simulink subsystem "AeroPropRefFranc"  (R2024b)
settings: Solver=VariableStepAuto  StartTime=0.0  StopTime=10.0  RelTol=1e-3
undefined symbols (not defined in the file or in its folder): ess, Force_b, Fprop_r, geom, H_b, Hdot_b, Moment_b, mot, mot2, mot3, mot4, Mprop_r, propel, propel2, propel3, propel4, pxf_diagram_options, SimIn, SimPar, tc, tc2, tc3, tc4
libraries: simulink x8, slpidlib x4, starslibAxisTransformations x2, libAxisTransformations x2
(part 3 of 10)

== system AeroPropRefFranc/Propulsion and Aerodynamic Forces and Moments/S-Function/Battery Model/powerplant/mot4/plant ==
  aInport--1 : Inport
  inport-ctrl_bus-2 : Inport  Port=2
  in-effort-2 : Inport  Port=3
  in-flow-3 : Inport  Port=4
  Ground_1 : Ground
  Terminator_1 : Terminator
  mot4_plant_map_Pelec_funTW_volt_in : Subsystem
  parameter_out : Subsystem
  parameter_selection : Subsystem
  outport-system_info_bus : Outport
  outport-plant_bus : Outport  Port=2
  out-effort-7 : Outport  Port=3
  out-flow-8 : Outport  Port=4
  wires:
  Ground_1/1 -> parameter_selection/1(Inport_1)
  aInport--1/1 -> Terminator_1/1
  mot4_plant_map_Pelec_funTW_volt_in/8(mot_current_out) -> out-flow-8/1
  mot4_plant_map_Pelec_funTW_volt_in/7(mot_trq_out mot_inertia_out) -> out-effort-7/1
  in-flow-3/1 -> mot4_plant_map_Pelec_funTW_volt_in/3(spd)
  in-effort-2/1 -> mot4_plant_map_Pelec_funTW_volt_in/2(voltage)
  parameter_selection/1(outport-mot4_ctrl_cmd_simu-1) -> mot4_plant_map_Pelec_funTW_volt_in/1(mot_ctrl_cmd_simu)
  mot4_plant_map_Pelec_funTW_volt_in/6(mot_plant_temp_coeff_simu) -> parameter_out/6(inport-mot4_plant_temp_coeff_simu)
  mot4_plant_map_Pelec_funTW_volt_in/5(mot_plant_trq_out_simu) -> parameter_out/5(inport-mot4_plant_trq_out_simu)
  mot4_plant_map_Pelec_funTW_volt_in/4(mot_plant_cmd_simu) -> parameter_out/4(inport-mot4_plant_cmd_simu)
  mot4_plant_map_Pelec_funTW_volt_in/3(mot_plant_volt_in_simu) -> parameter_out/3(inport-mot4_plant_volt_in_simu)
  mot4_plant_map_Pelec_funTW_volt_in/2(mot_plant_curr_in_simu) -> parameter_out/2(inport-mot4_plant_curr_in_simu)
  mot4_plant_map_Pelec_funTW_volt_in/1(mot_plant_spd_out_simu) -> parameter_out/1(inport-mot4_plant_spd_out_simu)
  parameter_out/2(outport-plant_bus) -> outport-plant_bus/1
  parameter_out/1(outport-system_info_bus) -> outport-system_info_bus/1
  inport-ctrl_bus-2/1 -> parameter_selection/2(inport-ctrl_bus-2)

== system AeroPropRefFranc/Propulsion and Aerodynamic Forces and Moments/S-Function/Battery Model/powerplant/propel/plant ==
  inport-main_info_bus-1 : Inport
  aInport--2 : Inport  Port=2
  in-effort-4 : Inport  Port=3
  in-flow-5 : Inport  Port=4
  Ground_1 : Ground
  Terminator_1 : Terminator
  parameter_out : Subsystem
  parameter_selection : Subsystem
  propel_plant_uas : Subsystem
  outport-system_info_bus : Outport
  aOutport--2 : Outport  Port=2
  out-effort-5 : Outport  Port=3
  out-flow-6 : Outport  Port=4
  wires:
  Ground_1/1 -> aOutport--2/1
  aInport--2/1 -> Terminator_1/1
  propel_plant_uas/6(propel_plant_speed_out_simu) -> out-flow-6/1
  propel_plant_uas/5(propel_plant_effort) -> out-effort-5/1
  in-flow-5/1 -> propel_plant_uas/5(flow-in)
  in-effort-4/1 -> propel_plant_uas/4(tc_plant_trq_out_simu)
  parameter_selection/3(outport-eqnmotion_plant_linvel_simu-3) -> propel_plant_uas/3(eqnmotion_plant_linvel_simu)
  parameter_selection/2(outport-tc_plant_inertia_out_simu-2) -> propel_plant_uas/2(tc_plant_inertia_out_simu)
  parameter_selection/1(outport-env_plant_density_simu-1) -> propel_plant_uas/1(env_plant_density_simu)
  propel_plant_uas/4(propel_plant_thrust_simu) -> parameter_out/4(inport-propel_plant_thrust_simu)
  propel_plant_uas/3(propel_plant_pwr_out_simu) -> parameter_out/3(inport-propel_plant_pwr_out_simu)
  propel_plant_uas/2(propel_plant_pwr_in_simu) -> parameter_out/2(inport-propel_plant_pwr_in_simu)
  propel_plant_uas/1(propel_plant_speed_simu) -> parameter_out/1(inport-propel_plant_speed_simu)
  parameter_out/1(outport-system_info_bus) -> outport-system_info_bus/1
  inport-main_info_bus-1/1 -> parameter_selection/1(inport-main_info_bus-1)

== system AeroPropRefFranc/Propulsion and Aerodynamic Forces and Moments/S-Function/Battery Model/powerplant/propel2/plant ==
  inport-main_info_bus-1 : Inport
  aInport--2 : Inport  Port=2
  in-effort-4 : Inport  Port=3
  in-flow-5 : Inport  Port=4
  Ground_1 : Ground
  Terminator_1 : Terminator
  parameter_out : Subsystem
  parameter_selection : Subsystem
  propel2_plant_uas : Subsystem
  outport-system_info_bus : Outport
  aOutport--2 : Outport  Port=2
  out-effort-5 : Outport  Port=3
  out-flow-6 : Outport  Port=4
  wires:
  Ground_1/1 -> aOutport--2/1
  aInport--2/1 -> Terminator_1/1
  propel2_plant_uas/6(propel_plant_speed_out_simu) -> out-flow-6/1
  propel2_plant_uas/5(propel_plant_effort) -> out-effort-5/1
  in-flow-5/1 -> propel2_plant_uas/5(flow-in)
  in-effort-4/1 -> propel2_plant_uas/4(tc_plant_trq_out_simu)
  parameter_selection/3(outport-eqnmotion_plant_linvel_simu-3) -> propel2_plant_uas/3(eqnmotion_plant_linvel_simu)
  parameter_selection/2(outport-tc_plant_inertia_out_simu-2) -> propel2_plant_uas/2(tc_plant_inertia_out_simu)
  parameter_selection/1(outport-env_plant_density_simu-1) -> propel2_plant_uas/1(env_plant_density_simu)
  propel2_plant_uas/4(propel_plant_thrust_simu) -> parameter_out/4(inport-propel2_plant_thrust_simu)
  propel2_plant_uas/3(propel_plant_pwr_out_simu) -> parameter_out/3(inport-propel2_plant_pwr_out_simu)
  propel2_plant_uas/2(propel_plant_pwr_in_simu) -> parameter_out/2(inport-propel2_plant_pwr_in_simu)
  propel2_plant_uas/1(propel_plant_speed_simu) -> parameter_out/1(inport-propel2_plant_speed_simu)
  parameter_out/1(outport-system_info_bus) -> outport-system_info_bus/1
  inport-main_info_bus-1/1 -> parameter_selection/1(inport-main_info_bus-1)

== system AeroPropRefFranc/Propulsion and Aerodynamic Forces and Moments/S-Function/Battery Model/powerplant/propel3/plant ==
  inport-main_info_bus-1 : Inport
  aInport--2 : Inport  Port=2
  in-effort-4 : Inport  Port=3
  in-flow-5 : Inport  Port=4
  Ground_1 : Ground
  Terminator_1 : Terminator
  parameter_out : Subsystem
  parameter_selection : Subsystem
  propel3_plant_uas : Subsystem
  outport-system_info_bus : Outport
  aOutport--2 : Outport  Port=2
  out-effort-5 : Outport  Port=3
  out-flow-6 : Outport  Port=4
  wires:
  Ground_1/1 -> aOutport--2/1
  aInport--2/1 -> Terminator_1/1
  propel3_plant_uas/6(propel_plant_speed_out_simu) -> out-flow-6/1
  propel3_plant_uas/5(propel_plant_effort) -> out-effort-5/1
  in-flow-5/1 -> propel3_plant_uas/5(flow-in)
  in-effort-4/1 -> propel3_plant_uas/4(tc_plant_trq_out_simu)
  parameter_selection/3(outport-eqnmotion_plant_linvel_simu-3) -> propel3_plant_uas/3(eqnmotion_plant_linvel_simu)
  parameter_selection/2(outport-tc_plant_inertia_out_simu-2) -> propel3_plant_uas/2(tc_plant_inertia_out_simu)
  parameter_selection/1(outport-env_plant_density_simu-1) -> propel3_plant_uas/1(env_plant_density_simu)
  propel3_plant_uas/4(propel_plant_thrust_simu) -> parameter_out/4(inport-propel3_plant_thrust_simu)
  propel3_plant_uas/3(propel_plant_pwr_out_simu) -> parameter_out/3(inport-propel3_plant_pwr_out_simu)
  propel3_plant_uas/2(propel_plant_pwr_in_simu) -> parameter_out/2(inport-propel3_plant_pwr_in_simu)
  propel3_plant_uas/1(propel_plant_speed_simu) -> parameter_out/1(inport-propel3_plant_speed_simu)
  parameter_out/1(outport-system_info_bus) -> outport-system_info_bus/1
  inport-main_info_bus-1/1 -> parameter_selection/1(inport-main_info_bus-1)

== system AeroPropRefFranc/Propulsion and Aerodynamic Forces and Moments/S-Function/Battery Model/powerplant/propel4/plant ==
  inport-main_info_bus-1 : Inport
  aInport--2 : Inport  Port=2
  in-effort-4 : Inport  Port=3
  in-flow-5 : Inport  Port=4
  Ground_1 : Ground
  Terminator_1 : Terminator
  parameter_out : Subsystem
  parameter_selection : Subsystem
  propel4_plant_uas : Subsystem
  outport-system_info_bus : Outport
  aOutport--2 : Outport  Port=2
  out-effort-5 : Outport  Port=3
  out-flow-6 : Outport  Port=4
  wires:
  Ground_1/1 -> aOutport--2/1
  aInport--2/1 -> Terminator_1/1
  propel4_plant_uas/6(propel_plant_speed_out_simu) -> out-flow-6/1
  propel4_plant_uas/5(propel_plant_effort) -> out-effort-5/1
  in-flow-5/1 -> propel4_plant_uas/5(flow-in)
  in-effort-4/1 -> propel4_plant_uas/4(tc_plant_trq_out_simu)
  parameter_selection/3(outport-eqnmotion_plant_linvel_simu-3) -> propel4_plant_uas/3(eqnmotion_plant_linvel_simu)
  parameter_selection/2(outport-tc_plant_inertia_out_simu-2) -> propel4_plant_uas/2(tc_plant_inertia_out_simu)
  parameter_selection/1(outport-env_plant_density_simu-1) -> propel4_plant_uas/1(env_plant_density_simu)
  propel4_plant_uas/4(propel_plant_thrust_simu) -> parameter_out/4(inport-propel4_plant_thrust_simu)
  propel4_plant_uas/3(propel_plant_pwr_out_simu) -> parameter_out/3(inport-propel4_plant_pwr_out_simu)
  propel4_plant_uas/2(propel_plant_pwr_in_simu) -> parameter_out/2(inport-propel4_plant_pwr_in_simu)
  propel4_plant_uas/1(propel_plant_speed_simu) -> parameter_out/1(inport-propel4_plant_speed_simu)
  parameter_out/1(outport-system_info_bus) -> outport-system_info_bus/1
  inport-main_info_bus-1/1 -> parameter_selection/1(inport-main_info_bus-1)

== system AeroPropRefFranc/Propulsion and Aerodynamic Forces and Moments/S-Function/Battery Model/powerplant/tc/plant ==
  aInport--1 : Inport
  aInport--2 : Inport  Port=2
  in-effort-1 : Inport  Port=3
  in-flow-2 : Inport  Port=4
  Ground_1 : Ground
  Terminator_1 : Terminator
  Terminator_2 : Terminator
  parameter_out : Subsystem
  parameter_selection : Subsystem
  tc_plant_map_trqloss_funTW : Subsystem
  outport-system_info_bus : Outport
  aOutport--2 : Outport  Port=2
  out-effort-7 : Outport  Port=3
  out-flow-8 : Outport  Port=4
  wires:
  Ground_1/1 -> aOutport--2/1
  aInport--2/1 -> Terminator_2/1
  aInport--1/1 -> Terminator_1/1
  tc_plant_map_trqloss_funTW/8(tc_spd_in) -> out-flow-8/1
  tc_plant_map_trqloss_funTW/7(tc_trq_out) -> out-effort-7/1
  in-flow-2/1 -> tc_plant_map_trqloss_funTW/2(tc_spd_out)
  in-effort-1/1 -> tc_plant_map_trqloss_funTW/1(tc_trq_in tc_inertia_in)
  tc_plant_map_trqloss_funTW/6(tc_plant_inertia_out_simu) -> parameter_out/6(inport-tc_plant_inertia_out_simu)
  tc_plant_map_trqloss_funTW/5(tc_plant_inertia_in_simu) -> parameter_out/5(inport-tc_plant_inertia_in_simu)
  tc_plant_map_trqloss_funTW/4(tc_plant_spd_out_simu) -> parameter_out/4(inport-tc_plant_spd_out_simu)
  tc_plant_map_trqloss_funTW/3(tc_plant_spd_in_simu) -> parameter_out/3(inport-tc_plant_spd_in_simu)
  tc_plant_map_trqloss_funTW/2(tc_plant_trq_out_simu) -> parameter_out/2(inport-tc_plant_trq_out_simu)
  tc_plant_map_trqloss_funTW/1(tc_plant_trq_in_simu) -> parameter_out/1(inport-tc_plant_trq_in_simu)
  parameter_out/1(outport-system_info_bus) -> outport-system_info_bus/1

== system AeroPropRefFranc/Propulsion and Aerodynamic Forces and Moments/S-Function/Battery Model/powerplant/tc2/plant ==
  aInport--1 : Inport
  aInport--2 : Inport  Port=2
  in-effort-1 : Inport  Port=3
  in-flow-2 : Inport  Port=4
  Ground_1 : Ground
  Terminator_1 : Terminator
  Terminator_2 : Terminator
  parameter_out : Subsystem
  parameter_selection : Subsystem
  tc2_plant_map_trqloss_funTW : Subsystem
  outport-system_info_bus : Outport
  aOutport--2 : Outport  Port=2
  out-effort-7 : Outport  Port=3
  out-flow-8 : Outport  Port=4
  wires:
  Ground_1/1 -> aOutport--2/1
  aInport--2/1 -> Terminator_2/1
  aInport--1/1 -> Terminator_1/1
  tc2_plant_map_trqloss_funTW/8(tc_spd_in) -> out-flow-8/1
  tc2_plant_map_trqloss_funTW/7(tc_trq_out) -> out-effort-7/1
  in-flow-2/1 -> tc2_plant_map_trqloss_funTW/2(tc_spd_out)
  in-effort-1/1 -> tc2_plant_map_trqloss_funTW/1(tc_trq_in tc_inertia_in)
  tc2_plant_map_trqloss_funTW/6(tc_plant_inertia_out_simu) -> parameter_out/6(inport-tc2_plant_inertia_out_simu)
  tc2_plant_map_trqloss_funTW/5(tc_plant_inertia_in_simu) -> parameter_out/5(inport-tc2_plant_inertia_in_simu)
  tc2_plant_map_trqloss_funTW/4(tc_plant_spd_out_simu) -> parameter_out/4(inport-tc2_plant_spd_out_simu)
  tc2_plant_map_trqloss_funTW/3(tc_plant_spd_in_simu) -> parameter_out/3(inport-tc2_plant_spd_in_simu)
  tc2_plant_map_trqloss_funTW/2(tc_plant_trq_out_simu) -> parameter_out/2(inport-tc2_plant_trq_out_simu)
  tc2_plant_map_trqloss_funTW/1(tc_plant_trq_in_simu) -> parameter_out/1(inport-tc2_plant_trq_in_simu)
  parameter_out/1(outport-system_info_bus) -> outport-system_info_bus/1

== system AeroPropRefFranc/Propulsion and Aerodynamic Forces and Moments/S-Function/Battery Model/powerplant/tc3/plant ==
  aInport--1 : Inport
  aInport--2 : Inport  Port=2
  in-effort-1 : Inport  Port=3
  in-flow-2 : Inport  Port=4
  Ground_1 : Ground
  Terminator_1 : Terminator
  Terminator_2 : Terminator
  parameter_out : Subsystem
  parameter_selection : Subsystem
  tc3_plant_map_trqloss_funTW : Subsystem
  outport-system_info_bus : Outport
  aOutport--2 : Outport  Port=2
  out-effort-7 : Outport  Port=3
  out-flow-8 : Outport  Port=4
  wires:
  Ground_1/1 -> aOutport--2/1
  aInport--2/1 -> Terminator_2/1
  aInport--1/1 -> Terminator_1/1
  tc3_plant_map_trqloss_funTW/8(tc_spd_in) -> out-flow-8/1
  tc3_plant_map_trqloss_funTW/7(tc_trq_out) -> out-effort-7/1
  in-flow-2/1 -> tc3_plant_map_trqloss_funTW/2(tc_spd_out)
  in-effort-1/1 -> tc3_plant_map_trqloss_funTW/1(tc_trq_in tc_inertia_in)
  tc3_plant_map_trqloss_funTW/6(tc_plant_inertia_out_simu) -> parameter_out/6(inport-tc3_plant_inertia_out_simu)
  tc3_plant_map_trqloss_funTW/5(tc_plant_inertia_in_simu) -> parameter_out/5(inport-tc3_plant_inertia_in_simu)
  tc3_plant_map_trqloss_funTW/4(tc_plant_spd_out_simu) -> parameter_out/4(inport-tc3_plant_spd_out_simu)
  tc3_plant_map_trqloss_funTW/3(tc_plant_spd_in_simu) -> parameter_out/3(inport-tc3_plant_spd_in_simu)
  tc3_plant_map_trqloss_funTW/2(tc_plant_trq_out_simu) -> parameter_out/2(inport-tc3_plant_trq_out_simu)
  tc3_plant_map_trqloss_funTW/1(tc_plant_trq_in_simu) -> parameter_out/1(inport-tc3_plant_trq_in_simu)
  parameter_out/1(outport-system_info_bus) -> outport-system_info_bus/1

== system AeroPropRefFranc/Propulsion and Aerodynamic Forces and Moments/S-Function/Battery Model/powerplant/tc4/plant ==
  aInport--1 : Inport
  aInport--2 : Inport  Port=2
  in-effort-1 : Inport  Port=3
  in-flow-2 : Inport  Port=4
  Ground_1 : Ground
  Terminator_1 : Terminator
  Terminator_2 : Terminator
  parameter_out : Subsystem
  parameter_selection : Subsystem
  tc4_plant_map_trqloss_funTW : Subsystem
  outport-system_info_bus : Outport
  aOutport--2 : Outport  Port=2
  out-effort-7 : Outport  Port=3
  out-flow-8 : Outport  Port=4
  wires:
  Ground_1/1 -> aOutport--2/1
  aInport--2/1 -> Terminator_2/1
  aInport--1/1 -> Terminator_1/1
  tc4_plant_map_trqloss_funTW/8(tc_spd_in) -> out-flow-8/1
  tc4_plant_map_trqloss_funTW/7(tc_trq_out) -> out-effort-7/1
  in-flow-2/1 -> tc4_plant_map_trqloss_funTW/2(tc_spd_out)
  in-effort-1/1 -> tc4_plant_map_trqloss_funTW/1(tc_trq_in tc_inertia_in)
  tc4_plant_map_trqloss_funTW/6(tc_plant_inertia_out_simu) -> parameter_out/6(inport-tc4_plant_inertia_out_simu)
  tc4_plant_map_trqloss_funTW/5(tc_plant_inertia_in_simu) -> parameter_out/5(inport-tc4_plant_inertia_in_simu)
  tc4_plant_map_trqloss_funTW/4(tc_plant_spd_out_simu) -> parameter_out/4(inport-tc4_plant_spd_out_simu)
  tc4_plant_map_trqloss_funTW/3(tc_plant_spd_in_simu) -> parameter_out/3(inport-tc4_plant_spd_in_simu)
  tc4_plant_map_trqloss_funTW/2(tc_plant_trq_out_simu) -> parameter_out/2(inport-tc4_plant_trq_out_simu)
  tc4_plant_map_trqloss_funTW/1(tc_plant_trq_in_simu) -> parameter_out/1(inport-tc4_plant_trq_in_simu)
  parameter_out/1(outport-system_info_bus) -> outport-system_info_bus/1

== system AeroPropRefFranc/Propulsion and Aerodynamic Forces and Moments/S-Function/Battery Model/ess (battery)/ctrl/ess_ctrl_pngv_map_anl_PI_cstr/PI controller for maximal charge power and current1 ==
  ess voltage : Inport
  ess curr : Inport  Port=2
  SOC : Inport  Port=3
  Burst maximal power : Lookup  InputValues=ess.plant.init.pwr_chg_10sec.idx1_soc  Table=ess.plant.init.pwr_chg_10sec.map  SaturateOnIntegerOverflow=off
  Continuous maximal power : Lookup  InputValues=ess.plant.init.pwr_chg.idx1_soc  Table=ess.plant.init.pwr_chg.map  SaturateOnIntegerOverflow=off
  Interpolation (curr) : Fcn  Expr=u(3)*u(1) + u(2)*(1-u(1))
  Interpolation (curr)1 : Fcn  Expr=u(3)*u(1) + u(2)*(1-u(1))
  Mux1 : Mux  Inputs=3
  Mux2 : Mux  Inputs=3
  "PI Ratio Calculator (curr) " : Subsystem
  PI Ratio Calculator (curr) 1 : Subsystem
  Product : Product  RndMeth=Zero
  Saturation : Saturate  UpperLimit=0  LowerLimit=-inf
  Saturation1 : Saturate  UpperLimit=0  LowerLimit=-inf
  "ess curr " : InportShadow  Port=2
  ess maximum current (burst charge) : Lookup  InputValues=ess.plant.init.curr_chg_burst_max.idx1_soc  Table=ess.plant.init.curr_chg_burst_max.map  SaturateOnIntegerOverflow=off
  ess maximum current (continuous charge) : Lookup  InputValues=ess.plant.init.curr_chg_cont_max.idx1_soc  Table=ess.plant.init.curr_chg_cont_max.map  SaturateOnIntegerOverflow=off
  ess.init.num_cell1 : Gain  Gain=ess.plant.init.num_cell  SaturateOnIntegerOverflow=on  OutDataTypeStr=Inherit: Same as input  ParamDataTypeStr=Inherit: Same as input
  ess.init.num_cell2 : Gain  Gain=ess.plant.init.num_cell  SaturateOnIntegerOverflow=on  OutDataTypeStr=Inherit: Same as input  ParamDataTypeStr=Inherit: Same as input
  ess.init.num_module_parallel1 : Gain  Gain=ess.plant.init.num_module_parallel
  ess.init.num_module_parallel5 : Gain  Gain=ess.plant.init.num_module_parallel
  Pwr_max_reg : Outport
  Curr_max_reg : Outport  Port=2
  wires:
  Saturation/1 -> "PI Ratio Calculator (curr) "/1(ess curr)
  "PI Ratio Calculator (curr) "/1(Current ratio) -> Mux1/1
  ess maximum current (burst charge)/1 -> ess.init.num_module_parallel1/1
  ess maximum current (continuous charge)/1 -> ess.init.num_module_parallel5/1
  ess curr/1 -> Saturation/1
  Mux1/1 -> Interpolation (curr)/1
  Interpolation (curr)/1 -> Curr_max_reg/1
  SOC/1 -> Continuous maximal power/1, Burst maximal power/1, ess maximum current (continuous charge)/1, ess maximum current (burst charge)/1
  Saturation1/1 -> PI Ratio Calculator (curr) 1/1(ess pwr)
  Continuous maximal power/1 -> ess.init.num_cell2/1
  Interpolation (curr)1/1 -> Pwr_max_reg/1
  Mux2/1 -> Interpolation (curr)1/1
  PI Ratio Calculator (curr) 1/1(pwr ratio) -> Mux2/1
  Burst maximal power/1 -> ess.init.num_cell1/1
  "ess curr "/1 -> Product/2
  ess voltage/1 -> Product/1
  Product/1 -> Saturation1/1
  ess.init.num_cell2/1 -> Mux2/2, PI Ratio Calculator (curr) 1/2(pwr max cont)
  ess.init.num_cell1/1 -> Mux2/3
  ess.init.num_module_parallel5/1 -> Mux1/2, "PI Ratio Calculator (curr) "/2(curr max cont)
  ess.init.num_module_parallel1/1 -> Mux1/3

== system AeroPropRefFranc/Propulsion and Aerodynamic Forces and Moments/S-Function/Battery Model/ess (battery)/ctrl/ess_ctrl_pngv_map_anl_PI_cstr/PI controller for maximal discharge power and current1 ==
  ess voltage : Inport
  ess curr : Inport  Port=2
  SOC : Inport  Port=3
  Burst maximal power : Lookup  InputValues=ess.plant.init.pwr_dis_10sec.idx1_soc  Table=ess.plant.init.pwr_dis_10sec.map  SaturateOnIntegerOverflow=off
  Continuous maximal power : Lookup  InputValues=ess.plant.init.pwr_dis.idx1_soc  Table=ess.plant.init.pwr_dis.map  SaturateOnIntegerOverflow=off
  Interpolation (curr) : Fcn  Expr=u(3)*u(1) + u(2)*(1-u(1))
  Interpolation (curr)1 : Fcn  Expr=u(3)*u(1) + u(2)*(1-u(1))
  Mux1 : Mux  Inputs=3
  Mux2 : Mux  Inputs=3
  "PI Ratio Calculator (curr) " : Subsystem
  PI Ratio Calculator (curr) 1 : Subsystem
  Product : Product  RndMeth=Zero
  Saturation : Saturate  UpperLimit=inf  LowerLimit=0
  Saturation1 : Saturate  UpperLimit=inf  LowerLimit=0
  "ess curr " : InportShadow  Port=2
  ess maximum current (burst discharge)1 : Lookup  InputValues=ess.plant.init.curr_dis_burst_max.idx1_soc  Table=ess.plant.init.curr_dis_burst_max.map  SaturateOnIntegerOverflow=off
  "ess maximum current (continuous discharge) " : Lookup  InputValues=ess.plant.init.curr_dis_cont_max.idx1_soc  Table=ess.plant.init.curr_dis_cont_max.map  SaturateOnIntegerOverflow=off
  ess.init.num_cell1 : Gain  Gain=ess.plant.init.num_cell  SaturateOnIntegerOverflow=on  OutDataTypeStr=Inherit: Same as input  ParamDataTypeStr=Inherit: Same as input
  ess.init.num_cell2 : Gain  Gain=ess.plant.init.num_cell  SaturateOnIntegerOverflow=on  OutDataTypeStr=Inherit: Same as input  ParamDataTypeStr=Inherit: Same as input
  ess.init.num_module_parallel1 : Gain  Gain=ess.plant.init.num_module_parallel
  ess.init.num_module_parallel5 : Gain  Gain=ess.plant.init.num_module_parallel
  Curr_max_prop : Outport
  Pwr_max_prop : Outport  Port=2
  wires:
  Interpolation (curr)/1 -> Curr_max_prop/1
  Mux1/1 -> Interpolation (curr)/1
  ess curr/1 -> Saturation/1
  "ess maximum current (continuous discharge) "/1 -> ess.init.num_module_parallel5/1
  ess maximum current (burst discharge)1/1 -> ess.init.num_module_parallel1/1
  "PI Ratio Calculator (curr) "/1(Current ratio) -> Mux1/1
  Saturation/1 -> "PI Ratio Calculator (curr) "/1(ess curr)
  SOC/1 -> Continuous maximal power/1, Burst maximal power/1, "ess maximum current (continuous discharge) "/1, ess maximum current (burst discharge)1/1
  Saturation1/1 -> PI Ratio Calculator (curr) 1/1(ess pwr)
  Continuous maximal power/1 -> ess.init.num_cell1/1
  Interpolation (curr)1/1 -> Pwr_max_prop/1
  Mux2/1 -> Interpolation (curr)1/1
  PI Ratio Calculator (curr) 1/1(pwr ratio) -> Mux2/1
  Burst maximal power/1 -> ess.init.num_cell2/1
  "ess curr "/1 -> Product/2
  ess voltage/1 -> Product/1
  Product/1 -> Saturation1/1
  ess.init.num_cell1/1 -> Mux2/2, PI Ratio Calculator (curr) 1/2(pwr max cont)
  ess.init.num_cell2/1 -> Mux2/3
  ess.init.num_module_parallel5/1 -> "PI Ratio Calculator (curr) "/2(curr max cont), Mux1/2
  ess.init.num_module_parallel1/1 -> Mux1/3

== system AeroPropRefFranc/Propulsion and Aerodynamic Forces and Moments/S-Function/Battery Model/ess (battery)/plant/ess_plant_pngv_map_anl_PI_cstr/ess_cell ==
  ess_cell_curr : Inport
  Memory : Memory
  current polarization : Subsystem
  current polarization1 : Subsystem
  ess_soc_calculation : Subsystem
  voltage calculation : Subsystem
  ess_cell_volt_out : Outport
  ess_cell_soc : Outport  Port=2
  ess_cell_voc : Outport  Port=3
  ess_cell_rint : Outport  Port=4
  ess_cell_rpol1 : Outport  Port=5
  ess_cell_rpol2 : Outport  Port=6
  ess_cell_curr_polar2 : Outport  Port=7
  ess_cell_curr_polar1 : Outport  Port=8
  wires:
  current polarization/1(ess_cell_curr_polar1) -> ess_cell_curr_polar1/1, voltage calculation/3(ess_cell_curr_pol1)
  Memory/1 -> voltage calculation/2(ess_cell_curr), current polarization/2(ess curr), current polarization1/2(ess curr), ess_soc_calculation/1(cell_curr)
  ess_soc_calculation/1(ess_soc) -> current polarization/1(ess soc), ess_cell_soc/1, voltage calculation/1(absolute SOC), current polarization1/1(ess soc)
  current polarization1/1(ess_cell_curr_polar2) -> ess_cell_curr_polar2/1, voltage calculation/4(ess_cell_curr_plo2)
  voltage calculation/1(ess_cell_volt) -> ess_cell_volt_out/1
  voltage calculation/2(ess_cell_voc) -> ess_cell_voc/1
  voltage calculation/3(ess_cell_rint) -> ess_cell_rint/1
  voltage calculation/4(ess_cell_rpol1) -> ess_cell_rpol1/1
  voltage calculation/5(ess_cell_rpol2) -> ess_cell_rpol2/1
  ess_cell_curr/1 -> Memory/1

== system AeroPropRefFranc/Propulsion and Aerodynamic Forces and Moments/S-Function/Battery Model/ess (battery)/plant/ess_plant_pngv_map_anl_PI_cstr/heat_generated ==
  volt_out : Inport
  ocv : Inport  Port=2
  load_current : Inport  Port=3
  Add : Sum  Inputs=-+
  Divide : Product  Inputs=*/
  Memory : Memory  InitialCondition=eps
  Product : Product  RndMeth=Zero
  square : Math  Operator=square  SignedPower=on
  heat_J : Outport
  impedance : Outport  Port=2
  wires:
  volt_out/1 -> Add/1
  ocv/1 -> Add/2
  load_current/1 -> Memory/1
  square/1 -> Product/2  "I sq"
  Product/1 -> heat_J/1
  Add/1 -> Divide/1
  Divide/1 -> Product/1, impedance/1  "R"
  Memory/1 -> square/1, Divide/2

== system AeroPropRefFranc/Propulsion and Aerodynamic Forces and Moments/S-Function/Battery Model/powerplant/accelec/plant/accelec_plant_const_pwrloss_volt_in_nokey ==
  drv_key_on_dmd_simu : Inport
  accelec_volt_in : Inport  Port=2
  accelec_curr_out : Inport  Port=3
  Electrical Power : Constant  Value=accelec.plant.init.pwr
  Product : Product  Inputs=*/  InputSameDT=on  SaturateOnIntegerOverflow=on  OutDataTypeStr=Inherit: Same as first input
  Sum : Sum  InputSameDT=on  SaturateOnIntegerOverflow=on  OutDataTypeStr=Inherit: Same as first input
  Sum1 : Sum  InputSameDT=on  SaturateOnIntegerOverflow=on  OutDataTypeStr=Inherit: Same as first input
  Terminator : Terminator
  eps : Constant  Value=eps
  accelec_plant_volt_in_simu : Outport  VectorParamsAs1DForOutWhenUnconnected=off
  accelec_plant_pwr_simu : Outport  Port=2  VectorParamsAs1DForOutWhenUnconnected=off
  accelec_plant_curr_in_simu : Outport  Port=3  VectorParamsAs1DForOutWhenUnconnected=off
  accelec_plant_volt_out_simu : Outport  Port=4  VectorParamsAs1DForOutWhenUnconnected=off
  accelec_plant_curr_out_simu : Outport  Port=5  VectorParamsAs1DForOutWhenUnconnected=off
  accelec_volt_out : Outport  Port=6  VectorParamsAs1DForOutWhenUnconnected=off
  accelec_curr_in : Outport  Port=7  VectorParamsAs1DForOutWhenUnconnected=off
  wires:
  [accelec_plant_pwr_simu] -> accelec_plant_pwr_simu/1  "accelec_plant_pwr_simu"
  accelec_volt_in/1 -> Sum1/1, [accelec_plant_volt_in_simu], [accelec_plant_volt_out_simu], accelec_volt_out/1
  [accelec_plant_volt_in_simu] -> accelec_plant_volt_in_simu/1  "accelec_plant_volt_in_simu"
  eps/1 -> Sum1/2
  Product/1 -> [accelec_plant_curr_simu], Sum/1
  accelec_curr_out/1 -> [accelec_plant_curr_out_simu], Sum/2
  Sum/1 -> [accelec_plant_curr_in_simu], accelec_curr_in/1
  Sum1/1 -> Product/2
  [accelec_plant_curr_in_simu] -> accelec_plant_curr_in_simu/1  "accelec_plant_curr_in_simu"
  [accelec_plant_curr_out_simu] -> accelec_plant_curr_out_simu/1  "accelec_plant_curr_out_simu"
  [accelec_plant_volt_out_simu] -> accelec_plant_volt_out_simu/1  "accelec_plant_volt_out_simu"
  Electrical Power/1 -> [accelec_plant_pwr_simu], Product/1
  drv_key_on_dmd_simu/1 -> Terminator/1

== system AeroPropRefFranc/Propulsion and Aerodynamic Forces and Moments/S-Function/Battery Model/powerplant/accelec/plant/parameter_out ==
  inport-accelec_plant_volt_in_simu : Inport
  inport-accelec_plant_pwr_simu : Inport  Port=2
  inport-accelec_plant_curr_in_simu : Inport  Port=3
  inport-accelec_plant_volt_out_simu : Inport  Port=4
  inport-accelec_plant_curr_out_simu : Inport  Port=5
  Ground_1 : Ground
  Toworkspace-accelec_plant_curr_in_simu : ToWorkspace  VariableName=accelec_plant_curr_in_simu  SampleTime=pxf_diagram_options.workspace_sample_time
      settings: Decimation=pxf_diagram_options.decimation
  Toworkspace-accelec_plant_curr_out_simu : ToWorkspace  VariableName=accelec_plant_curr_out_simu  SampleTime=pxf_diagram_options.workspace_sample_time
      settings: Decimation=pxf_diagram_options.decimation
  Toworkspace-accelec_plant_pwr_simu : ToWorkspace  VariableName=accelec_plant_pwr_simu  SampleTime=pxf_diagram_options.workspace_sample_time
      settings: Decimation=pxf_diagram_options.decimation
  Toworkspace-accelec_plant_volt_in_simu : ToWorkspace  VariableName=accelec_plant_volt_in_simu  SampleTime=pxf_diagram_options.workspace_sample_time
      settings: Decimation=pxf_diagram_options.decimation
  Toworkspace-accelec_plant_volt_out_simu : ToWorkspace  VariableName=accelec_plant_volt_out_simu  SampleTime=pxf_diagram_options.workspace_sample_time
      settings: Decimation=pxf_diagram_options.decimation
  outport-system_info_bus : Outport
  wires:
  Ground_1/1 -> outport-system_info_bus/1
  inport-accelec_plant_curr_out_simu/1 -> Toworkspace-accelec_plant_curr_out_simu/1
  inport-accelec_plant_volt_out_simu/1 -> Toworkspace-accelec_plant_volt_out_simu/1
  inport-accelec_plant_curr_in_simu/1 -> Toworkspace-accelec_plant_curr_in_simu/1
  inport-accelec_plant_pwr_simu/1 -> Toworkspace-accelec_plant_pwr_simu/1
  inport-accelec_plant_volt_in_simu/1 -> Toworkspace-accelec_plant_volt_in_simu/1

== system AeroPropRefFranc/Propulsion and Aerodynamic Forces and Moments/S-Function/Battery Model/powerplant/accelec/plant/parameter_selection ==

== system AeroPropRefFranc/Propulsion and Aerodynamic Forces and Moments/S-Function/Battery Model/powerplant/ess (battery)/ctrl/ess_ctrl_pngv_map_anl_PI_cstr ==
  ess_volt_out : Inport
  ess_curr_out : Inport  Port=2
  ess_soc : Inport  Port=3
  Demux : Demux  Outputs=3
  Demux1 : Demux  Outputs=3
  PI controller for maximal charge power and current1 : Subsystem
  PI controller for maximal discharge power and current1 : Subsystem
  mux1 : Mux  Inputs=3
  ess_ctrl_pwr_max_pro_simu : Outport
  ess_ctrl_pwr_max_reg_simu : Outport  Port=2
  ess_ctrl_curr_max_pro_simu : Outport  Port=3
  ess_ctrl_curr_max_reg_simu : Outport  Port=4
  wires:
  [ess_ctrl_pwr_max_reg_simu] -> ess_ctrl_pwr_max_reg_simu/1  "ess_ctrl_pwr_max_reg_simu"
  [ess_ctrl_pwr_max_pro_simu] -> ess_ctrl_pwr_max_pro_simu/1  "ess_ctrl_pwr_max_pro_simu"
  [ess_ctrl_curr_max_pro_simu] -> ess_ctrl_curr_max_pro_simu/1  "ess_ctrl_curr_max_pro_simu"
  [ess_ctrl_curr_max_reg_simu] -> ess_ctrl_curr_max_reg_simu/1  "ess_ctrl_curr_max_reg_simu"
  PI controller for maximal discharge power and current1/1(Curr_max_prop) -> [ess_ctrl_curr_max_pro_simu]
  PI controller for maximal charge power and current1/2(Curr_max_reg) -> [ess_ctrl_curr_max_reg_simu]
  ess_volt_out/1 -> mux1/1  "ess_plant_volt_out_simu"
  mux1/1 -> Demux/1, Demux1/1
  PI controller for maximal discharge power and current1/2(Pwr_max_prop) -> [ess_ctrl_pwr_max_pro_simu]
  PI controller for maximal charge power and current1/1(Pwr_max_reg) -> [ess_ctrl_pwr_max_reg_simu]
  Demux/1 -> PI controller for maximal discharge power and current1/1(ess voltage)
  Demux/2 -> PI controller for maximal discharge power and current1/2(ess curr)
  Demux/3 -> PI controller for maximal discharge power and current1/3(SOC)
  Demux1/1 -> PI controller for maximal charge power and current1/1(ess voltage)
  Demux1/2 -> PI controller for maximal charge power and current1/2(ess curr)
  Demux1/3 -> PI controller for maximal charge power and current1/3(SOC)
  ess_curr_out/1 -> mux1/2  "ess_plant_curr_out_simu"
  ess_soc/1 -> mux1/3  "ess_plant_soc_simu"

== system AeroPropRefFranc/Propulsion and Aerodynamic Forces and Moments/S-Function/Battery Model/powerplant/ess (battery)/ctrl/parameter_out ==
  inport-ess_ctrl_pwr_max_pro_simu : Inport
  inport-ess_ctrl_pwr_max_reg_simu : Inport  Port=2
  inport-ess_ctrl_curr_max_pro_simu : Inport  Port=3
  inport-ess_ctrl_curr_max_reg_simu : Inport  Port=4
  Ground_1 : Ground
  Toworkspace-ess_ctrl_curr_max_pro_simu : ToWorkspace  VariableName=ess_ctrl_curr_max_pro_simu  SampleTime=pxf_diagram_options.workspace_sample_time
      settings: Decimation=pxf_diagram_options.decimation
  Toworkspace-ess_ctrl_curr_max_reg_simu : ToWorkspace  VariableName=ess_ctrl_curr_max_reg_simu  SampleTime=pxf_diagram_options.workspace_sample_time
      settings: Decimation=pxf_diagram_options.decimation
  Toworkspace-ess_ctrl_pwr_max_pro_simu : ToWorkspace  VariableName=ess_ctrl_pwr_max_pro_simu  SampleTime=pxf_diagram_options.workspace_sample_time
      settings: Decimation=pxf_diagram_options.decimation
  Toworkspace-ess_ctrl_pwr_max_reg_simu : ToWorkspace  VariableName=ess_ctrl_pwr_max_reg_simu  SampleTime=pxf_diagram_options.workspace_sample_time
      settings: Decimation=pxf_diagram_options.decimation
  create_system_info_bus : BusCreator  Inputs=1
  outport-system_info_bus : Outport
  outport-ctrl_bus : Outport  Port=2
  wires:
  Ground_1/1 -> outport-ctrl_bus/1
  inport-ess_ctrl_curr_max_reg_simu/1 -> Toworkspace-ess_ctrl_curr_max_reg_simu/1
  inport-ess_ctrl_curr_max_pro_simu/1 -> Toworkspace-ess_ctrl_curr_max_pro_simu/1
  inport-ess_ctrl_pwr_max_reg_simu/1 -> Toworkspace-ess_ctrl_pwr_max_reg_simu/1
  inport-ess_ctrl_pwr_max_pro_simu/1 -> Toworkspace-ess_ctrl_pwr_max_pro_simu/1, create_system_info_bus/1  "ess_ctrl_pwr_max_pro_simu"
  create_system_info_bus/1 -> outport-system_info_bus/1

== system AeroPropRefFranc/Propulsion and Aerodynamic Forces and Moments/S-Function/Battery Model/powerplant/ess (battery)/ctrl/parameter_selection ==
  inport-main_info_bus-1 : Inport
  select_main_info_bus : BusSelector  OutputSignals=apa_info_bus.powerplant_info_bus.ess.plant.ess_plant_volt_out_simu,apa_info_bus.powerplant_info_bus.ess.plant.ess_plant_curr_out_simu,apa_info_bus.powerplant_info_bus.ess.plant.ess_plant_soc_simu
  outport-ess_plant_volt_out_simu-1 : Outport
  outport-ess_plant_curr_out_simu-2 : Outport  Port=2
  outport-ess_plant_soc_simu-3 : Outport  Port=3
  wires:
  select_main_info_bus/3 -> outport-ess_plant_soc_simu-3/1  "<ess_plant_soc_simu>"
  select_main_info_bus/2 -> outport-ess_plant_curr_out_simu-2/1  "<ess_plant_curr_out_simu>"
  select_main_info_bus/1 -> outport-ess_plant_volt_out_simu-1/1  "<ess_plant_volt_out_simu>"
  inport-main_info_bus-1/1 -> select_main_info_bus/1

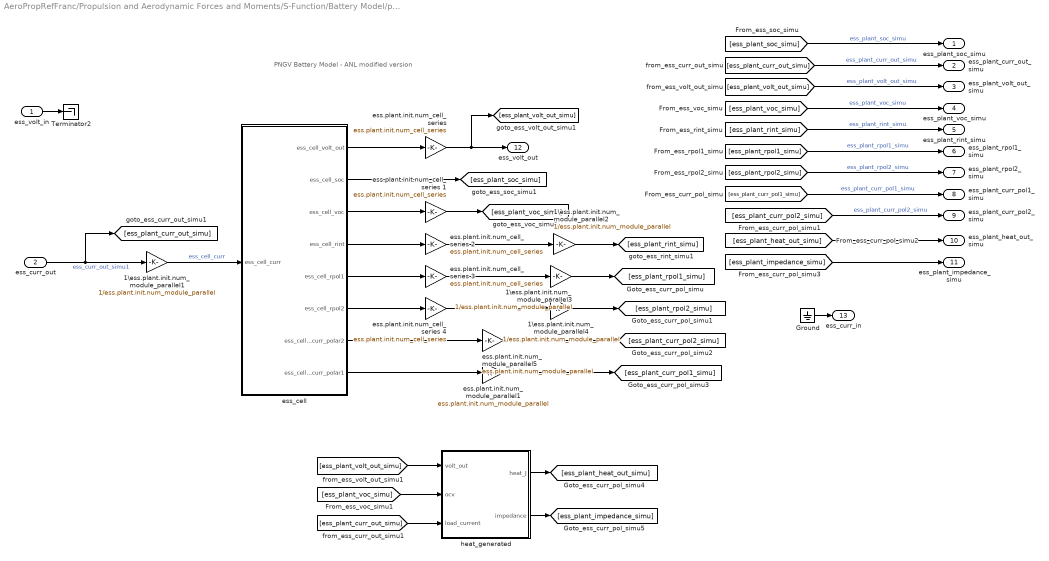
== system AeroPropRefFranc/Propulsion and Aerodynamic Forces and Moments/S-Function/Battery Model/powerplant/ess (battery)/plant/ess_plant_pngv_map_anl_PI_cstr ==
  note: PNGV Battery Model - ANL modified version
  ess_volt_in : Inport
  ess_curr_out : Inport  Port=2
  1\ess.plant.init.num_module_parallel{1..4} (4 alike) : Gain  Gain=1/ess.plant.init.num_module_parallel
  Ground : Ground
  Terminator2 : Terminator
  ess.plant.init.num_cell_series {,1..4} (5 alike) : Gain  Gain=ess.plant.init.num_cell_series
  ess.plant.init.num_module_parallel1 : Gain  Gain=ess.plant.init.num_module_parallel
  ess.plant.init.num_module_parallel5 : Gain  Gain=ess.plant.init.num_module_parallel
  ess_cell : Subsystem
  heat_generated : Subsystem
  ess_plant_soc_simu : Outport
  ess_plant_curr_out_simu : Outport  Port=2
  ess_plant_volt_out_simu : Outport  Port=3
  ess_plant_voc_simu : Outport  Port=4
  ess_plant_rint_simu : Outport  Port=5
  ess_plant_rpol1_simu : Outport  Port=6
  ess_plant_rpol2_simu : Outport  Port=7
  ess_plant_curr_pol1_simu : Outport  Port=8
  ess_plant_curr_pol2_simu : Outport  Port=9
  ess_plant_heat_out_simu : Outport  Port=10
  ess_plant_impedance_simu : Outport  Port=11
  ess_volt_out : Outport  Port=12
  ess_curr_in : Outport  Port=13
  wires:
  Ground/1 -> ess_curr_in/1
  ess_volt_in/1 -> Terminator2/1
  [ess_plant_soc_simu] -> ess_plant_soc_simu/1  "ess_plant_soc_simu"
  [ess_plant_curr_out_simu] -> ess_plant_curr_out_simu/1  "ess_plant_curr_out_simu"
  [ess_plant_volt_out_simu] -> ess_plant_volt_out_simu/1  "ess_plant_volt_out_simu"
  [ess_plant_voc_simu] -> ess_plant_voc_simu/1  "ess_plant_voc_simu"
  [ess_plant_rint_simu] -> ess_plant_rint_simu/1  "ess_plant_rint_simu"
  [ess_plant_rpol1_simu] -> ess_plant_rpol1_simu/1  "ess_plant_rpol1_simu"
  [ess_plant_rpol2_simu] -> ess_plant_rpol2_simu/1  "ess_plant_rpol2_simu"
  [ess_plant_curr_pol1_simu] -> ess_plant_curr_pol1_simu/1  "ess_plant_curr_pol1_simu"
  [ess_plant_curr_pol2_simu] -> ess_plant_curr_pol2_simu/1  "ess_plant_curr_pol2_simu"
  ess_cell/1(ess_cell_volt_out) -> "ess.plant.init.num_cell_series "/1
  1\ess.plant.init.num_module_parallel1/1 -> ess_cell/1(ess_cell_curr)  "ess_cell_curr"
  "ess.plant.init.num_cell_series "/1 -> [ess_plant_volt_out_simu], ess_volt_out/1
  ess.plant.init.num_cell_series 2/1 -> 1\ess.plant.init.num_module_parallel2/1
  ess.plant.init.num_cell_series 1/1 -> [ess_plant_voc_simu]
  1\ess.plant.init.num_module_parallel2/1 -> [ess_plant_rint_simu]
  ess_curr_out/1 -> 1\ess.plant.init.num_module_parallel1/1, [ess_plant_curr_out_simu]  "ess_curr_out_simu1"
  ess_cell/3(ess_cell_voc) -> ess.plant.init.num_cell_series 1/1
  ess_cell/4(ess_cell_rint) -> ess.plant.init.num_cell_series 2/1
  ess_cell/2(ess_cell_soc) -> [ess_plant_soc_simu]
  ess_cell/5(ess_cell_rpol1) -> ess.plant.init.num_cell_series 3/1
  ess_cell/6(ess_cell_rpol2) -> ess.plant.init.num_cell_series 4/1
  ess.plant.init.num_cell_series 3/1 -> 1\ess.plant.init.num_module_parallel3/1
  1\ess.plant.init.num_module_parallel3/1 -> [ess_plant_rpol1_simu]
  ess.plant.init.num_cell_series 4/1 -> 1\ess.plant.init.num_module_parallel4/1
  1\ess.plant.init.num_module_parallel4/1 -> [ess_plant_rpol2_simu]
  ess_cell/8(ess_cell_curr_polar1) -> ess.plant.init.num_module_parallel1/1
  ess_cell/7(ess_cell_curr_polar2) -> ess.plant.init.num_module_parallel5/1
  ess.plant.init.num_module_parallel5/1 -> [ess_plant_curr_pol2_simu]
  ess.plant.init.num_module_parallel1/1 -> [ess_plant_curr_pol1_simu]
  [ess_plant_volt_out_simu] -> heat_generated/1(volt_out)
  [ess_plant_voc_simu] -> heat_generated/2(ocv)
  [ess_plant_curr_out_simu] -> heat_generated/3(load_current)
  heat_generated/1(heat_J) -> [ess_plant_heat_out_simu]
  [ess_plant_heat_out_simu] -> ess_plant_heat_out_simu/1
  heat_generated/2(impedance) -> [ess_plant_impedance_simu]
  [ess_plant_impedance_simu] -> ess_plant_impedance_simu/1

== system AeroPropRefFranc/Propulsion and Aerodynamic Forces and Moments/S-Function/Battery Model/powerplant/ess (battery)/plant/parameter_out ==
  inport-ess_plant_soc_simu : Inport
  inport-ess_plant_curr_out_simu : Inport  Port=2
  inport-ess_plant_volt_out_simu : Inport  Port=3
  inport-ess_plant_voc_simu : Inport  Port=4
  inport-ess_plant_rint_simu : Inport  Port=5
  inport-ess_plant_rpol1_simu : Inport  Port=6
  inport-ess_plant_rpol2_simu : Inport  Port=7
  inport-ess_plant_curr_pol1_simu : Inport  Port=8
  inport-ess_plant_curr_pol2_simu : Inport  Port=9
  inport-ess_plant_heat_out_simu : Inport  Port=10
  inport-ess_plant_impedance_simu : Inport  Port=11
  Ground_1 : Ground
  Toworkspace-ess_plant_curr_out_simu : ToWorkspace  VariableName=ess_plant_curr_out_simu  SampleTime=pxf_diagram_options.workspace_sample_time
      settings: Decimation=pxf_diagram_options.decimation
  Toworkspace-ess_plant_curr_pol1_simu : ToWorkspace  VariableName=ess_plant_curr_pol1_simu  SampleTime=pxf_diagram_options.workspace_sample_time
      settings: Decimation=pxf_diagram_options.decimation
  Toworkspace-ess_plant_curr_pol2_simu : ToWorkspace  VariableName=ess_plant_curr_pol2_simu  SampleTime=pxf_diagram_options.workspace_sample_time
      settings: Decimation=pxf_diagram_options.decimation
  Toworkspace-ess_plant_heat_out_simu : ToWorkspace  VariableName=ess_plant_heat_out_simu  SampleTime=pxf_diagram_options.workspace_sample_time
      settings: Decimation=pxf_diagram_options.decimation
  Toworkspace-ess_plant_impedance_simu : ToWorkspace  VariableName=ess_plant_impedance_simu  SampleTime=pxf_diagram_options.workspace_sample_time
      settings: Decimation=pxf_diagram_options.decimation
  Toworkspace-ess_plant_rint_simu : ToWorkspace  VariableName=ess_plant_rint_simu  SampleTime=pxf_diagram_options.workspace_sample_time
      settings: Decimation=pxf_diagram_options.decimation
  Toworkspace-ess_plant_rpol1_simu : ToWorkspace  VariableName=ess_plant_rpol1_simu  SampleTime=pxf_diagram_options.workspace_sample_time
      settings: Decimation=pxf_diagram_options.decimation
  Toworkspace-ess_plant_rpol2_simu : ToWorkspace  VariableName=ess_plant_rpol2_simu  SampleTime=pxf_diagram_options.workspace_sample_time
      settings: Decimation=pxf_diagram_options.decimation
  Toworkspace-ess_plant_soc_simu : ToWorkspace  VariableName=ess_plant_soc_simu  SampleTime=pxf_diagram_options.workspace_sample_time
      settings: Decimation=pxf_diagram_options.decimation
  Toworkspace-ess_plant_voc_simu : ToWorkspace  VariableName=ess_plant_voc_simu  SampleTime=pxf_diagram_options.workspace_sample_time
      settings: Decimation=pxf_diagram_options.decimation
  Toworkspace-ess_plant_volt_out_simu : ToWorkspace  VariableName=ess_plant_volt_out_simu  SampleTime=pxf_diagram_options.workspace_sample_time
      settings: Decimation=pxf_diagram_options.decimation
  create_system_info_bus : BusCreator  Inputs=3
  outport-system_info_bus : Outport
  outport-plant_bus : Outport  Port=2
  wires:
  Ground_1/1 -> outport-plant_bus/1
  inport-ess_plant_curr_pol2_simu/1 -> Toworkspace-ess_plant_curr_pol2_simu/1
  inport-ess_plant_curr_pol1_simu/1 -> Toworkspace-ess_plant_curr_pol1_simu/1
  inport-ess_plant_rpol2_simu/1 -> Toworkspace-ess_plant_rpol2_simu/1
  inport-ess_plant_rpol1_simu/1 -> Toworkspace-ess_plant_rpol1_simu/1
  inport-ess_plant_rint_simu/1 -> Toworkspace-ess_plant_rint_simu/1
  inport-ess_plant_voc_simu/1 -> Toworkspace-ess_plant_voc_simu/1
  inport-ess_plant_volt_out_simu/1 -> Toworkspace-ess_plant_volt_out_simu/1, create_system_info_bus/3  "ess_plant_volt_out_simu"
  inport-ess_plant_curr_out_simu/1 -> Toworkspace-ess_plant_curr_out_simu/1, create_system_info_bus/2  "ess_plant_curr_out_simu"
  inport-ess_plant_impedance_simu/1 -> Toworkspace-ess_plant_impedance_simu/1
  inport-ess_plant_heat_out_simu/1 -> Toworkspace-ess_plant_heat_out_simu/1
  inport-ess_plant_soc_simu/1 -> Toworkspace-ess_plant_soc_simu/1, create_system_info_bus/1  "ess_plant_soc_simu"
  create_system_info_bus/1 -> outport-system_info_bus/1

== system AeroPropRefFranc/Propulsion and Aerodynamic Forces and Moments/S-Function/Battery Model/powerplant/ess (battery)/plant/parameter_selection ==

== system AeroPropRefFranc/Propulsion and Aerodynamic Forces and Moments/S-Function/Battery Model/powerplant/ess (battery)1/ctrl/ess_ctrl_pngv_map_anl_PI_cstr ==
  ess_volt_out : Inport
  ess_curr_out : Inport  Port=2
  ess_soc : Inport  Port=3
  Demux : Demux  Outputs=3
  Demux1 : Demux  Outputs=3
  PI controller for maximal charge power and current1 : Subsystem
  PI controller for maximal discharge power and current1 : Subsystem
  mux1 : Mux  Inputs=3
  ess_ctrl_pwr_max_pro_simu : Outport
  ess_ctrl_pwr_max_reg_simu : Outport  Port=2
  ess_ctrl_curr_max_pro_simu : Outport  Port=3
  ess_ctrl_curr_max_reg_simu : Outport  Port=4
  wires:
  ess_soc/1 -> mux1/3  "ess_plant_soc_simu"
  ess_curr_out/1 -> mux1/2  "ess_plant_curr_out_simu"
  Demux1/3 -> PI controller for maximal charge power and current1/3(SOC)
  Demux1/2 -> PI controller for maximal charge power and current1/2(ess curr)
  Demux1/1 -> PI controller for maximal charge power and current1/1(ess voltage)
  Demux/3 -> PI controller for maximal discharge power and current1/3(SOC)
  Demux/2 -> PI controller for maximal discharge power and current1/2(ess curr)
  Demux/1 -> PI controller for maximal discharge power and current1/1(ess voltage)
  PI controller for maximal charge power and current1/1(Pwr_max_reg) -> [ess_ctrl_pwr_max_reg_simu]
  PI controller for maximal discharge power and current1/2(Pwr_max_prop) -> [ess_ctrl_pwr_max_pro_simu]
  mux1/1 -> Demux1/1, Demux/1
  ess_volt_out/1 -> mux1/1  "ess_plant_volt_out_simu"
  PI controller for maximal charge power and current1/2(Curr_max_reg) -> [ess_ctrl_curr_max_reg_simu]
  PI controller for maximal discharge power and current1/1(Curr_max_prop) -> [ess_ctrl_curr_max_pro_simu]
  [ess_ctrl_curr_max_reg_simu] -> ess_ctrl_curr_max_reg_simu/1  "ess_ctrl_curr_max_reg_simu"
  [ess_ctrl_curr_max_pro_simu] -> ess_ctrl_curr_max_pro_simu/1  "ess_ctrl_curr_max_pro_simu"
  [ess_ctrl_pwr_max_pro_simu] -> ess_ctrl_pwr_max_pro_simu/1  "ess_ctrl_pwr_max_pro_simu"
  [ess_ctrl_pwr_max_reg_simu] -> ess_ctrl_pwr_max_reg_simu/1  "ess_ctrl_pwr_max_reg_simu"

== system AeroPropRefFranc/Propulsion and Aerodynamic Forces and Moments/S-Function/Battery Model/powerplant/ess (battery)1/ctrl/parameter_out ==
  inport-ess_ctrl_pwr_max_pro_simu : Inport
  inport-ess_ctrl_pwr_max_reg_simu : Inport  Port=2
  inport-ess_ctrl_curr_max_pro_simu : Inport  Port=3
  inport-ess_ctrl_curr_max_reg_simu : Inport  Port=4
  Ground_1 : Ground
  Toworkspace-ess_ctrl_curr_max_pro_simu : ToWorkspace  VariableName=ess_ctrl_curr_max_pro_simu  SampleTime=pxf_diagram_options.workspace_sample_time
      settings: Decimation=pxf_diagram_options.decimation
  Toworkspace-ess_ctrl_curr_max_reg_simu : ToWorkspace  VariableName=ess_ctrl_curr_max_reg_simu  SampleTime=pxf_diagram_options.workspace_sample_time
      settings: Decimation=pxf_diagram_options.decimation
  Toworkspace-ess_ctrl_pwr_max_pro_simu : ToWorkspace  VariableName=ess_ctrl_pwr_max_pro_simu  SampleTime=pxf_diagram_options.workspace_sample_time
      settings: Decimation=pxf_diagram_options.decimation
  Toworkspace-ess_ctrl_pwr_max_reg_simu : ToWorkspace  VariableName=ess_ctrl_pwr_max_reg_simu  SampleTime=pxf_diagram_options.workspace_sample_time
      settings: Decimation=pxf_diagram_options.decimation
  create_system_info_bus : BusCreator  Inputs=1
  outport-system_info_bus : Outport
  outport-ctrl_bus : Outport  Port=2
  wires:
  create_system_info_bus/1 -> outport-system_info_bus/1
  inport-ess_ctrl_pwr_max_pro_simu/1 -> create_system_info_bus/1, Toworkspace-ess_ctrl_pwr_max_pro_simu/1  "ess_ctrl_pwr_max_pro_simu"
  inport-ess_ctrl_pwr_max_reg_simu/1 -> Toworkspace-ess_ctrl_pwr_max_reg_simu/1
  inport-ess_ctrl_curr_max_pro_simu/1 -> Toworkspace-ess_ctrl_curr_max_pro_simu/1
  inport-ess_ctrl_curr_max_reg_simu/1 -> Toworkspace-ess_ctrl_curr_max_reg_simu/1
  Ground_1/1 -> outport-ctrl_bus/1

== system AeroPropRefFranc/Propulsion and Aerodynamic Forces and Moments/S-Function/Battery Model/powerplant/ess (battery)1/ctrl/parameter_selection ==
  inport-main_info_bus-1 : Inport
  select_main_info_bus : BusSelector  OutputSignals=apa_info_bus.powerplant_info_bus.ess.plant.ess_plant_volt_out_simu,apa_info_bus.powerplant_info_bus.ess.plant.ess_plant_curr_out_simu,apa_info_bus.powerplant_info_bus.ess.plant.ess_plant_soc_simu
  outport-ess_plant_volt_out_simu-1 : Outport
  outport-ess_plant_curr_out_simu-2 : Outport  Port=2
  outport-ess_plant_soc_simu-3 : Outport  Port=3
  wires:
  inport-main_info_bus-1/1 -> select_main_info_bus/1
  select_main_info_bus/1 -> outport-ess_plant_volt_out_simu-1/1  "<ess_plant_volt_out_simu>"
  select_main_info_bus/2 -> outport-ess_plant_curr_out_simu-2/1  "<ess_plant_curr_out_simu>"
  select_main_info_bus/3 -> outport-ess_plant_soc_simu-3/1  "<ess_plant_soc_simu>"

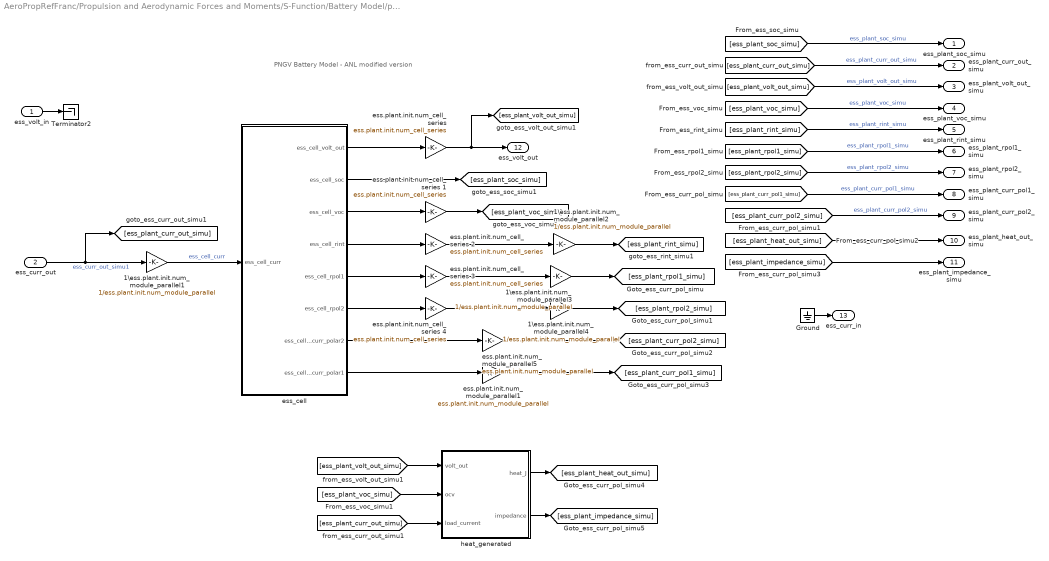
== system AeroPropRefFranc/Propulsion and Aerodynamic Forces and Moments/S-Function/Battery Model/powerplant/ess (battery)1/plant/ess_plant_pngv_map_anl_PI_cstr ==
  note: PNGV Battery Model - ANL modified version
  ess_volt_in : Inport
  ess_curr_out : Inport  Port=2
  1\ess.plant.init.num_module_parallel{1..4} (4 alike) : Gain  Gain=1/ess.plant.init.num_module_parallel
  Ground : Ground
  Terminator2 : Terminator
  ess.plant.init.num_cell_series {,1..4} (5 alike) : Gain  Gain=ess.plant.init.num_cell_series
  ess.plant.init.num_module_parallel1 : Gain  Gain=ess.plant.init.num_module_parallel
  ess.plant.init.num_module_parallel5 : Gain  Gain=ess.plant.init.num_module_parallel
  ess_cell : Subsystem
  heat_generated : Subsystem
  ess_plant_soc_simu : Outport
  ess_plant_curr_out_simu : Outport  Port=2
  ess_plant_volt_out_simu : Outport  Port=3
  ess_plant_voc_simu : Outport  Port=4
  ess_plant_rint_simu : Outport  Port=5
  ess_plant_rpol1_simu : Outport  Port=6
  ess_plant_rpol2_simu : Outport  Port=7
  ess_plant_curr_pol1_simu : Outport  Port=8
  ess_plant_curr_pol2_simu : Outport  Port=9
  ess_plant_heat_out_simu : Outport  Port=10
  ess_plant_impedance_simu : Outport  Port=11
  ess_volt_out : Outport  Port=12
  ess_curr_in : Outport  Port=13
  wires:
  [ess_plant_impedance_simu] -> ess_plant_impedance_simu/1
  heat_generated/2(impedance) -> [ess_plant_impedance_simu]
  [ess_plant_heat_out_simu] -> ess_plant_heat_out_simu/1
  heat_generated/1(heat_J) -> [ess_plant_heat_out_simu]
  [ess_plant_curr_out_simu] -> heat_generated/3(load_current)
  [ess_plant_voc_simu] -> heat_generated/2(ocv)
  [ess_plant_volt_out_simu] -> heat_generated/1(volt_out)
  ess.plant.init.num_module_parallel1/1 -> [ess_plant_curr_pol1_simu]
  ess.plant.init.num_module_parallel5/1 -> [ess_plant_curr_pol2_simu]
  ess_cell/7(ess_cell_curr_polar2) -> ess.plant.init.num_module_parallel5/1
  ess_cell/8(ess_cell_curr_polar1) -> ess.plant.init.num_module_parallel1/1
  1\ess.plant.init.num_module_parallel4/1 -> [ess_plant_rpol2_simu]
  ess.plant.init.num_cell_series 4/1 -> 1\ess.plant.init.num_module_parallel4/1
  1\ess.plant.init.num_module_parallel3/1 -> [ess_plant_rpol1_simu]
  ess.plant.init.num_cell_series 3/1 -> 1\ess.plant.init.num_module_parallel3/1
  ess_cell/6(ess_cell_rpol2) -> ess.plant.init.num_cell_series 4/1
  ess_cell/5(ess_cell_rpol1) -> ess.plant.init.num_cell_series 3/1
  ess_cell/2(ess_cell_soc) -> [ess_plant_soc_simu]
  ess_cell/4(ess_cell_rint) -> ess.plant.init.num_cell_series 2/1
  ess_cell/3(ess_cell_voc) -> ess.plant.init.num_cell_series 1/1
  ess_curr_out/1 -> [ess_plant_curr_out_simu], 1\ess.plant.init.num_module_parallel1/1  "ess_curr_out_simu1"
  1\ess.plant.init.num_module_parallel2/1 -> [ess_plant_rint_simu]
  ess.plant.init.num_cell_series 1/1 -> [ess_plant_voc_simu]
  ess.plant.init.num_cell_series 2/1 -> 1\ess.plant.init.num_module_parallel2/1
  "ess.plant.init.num_cell_series "/1 -> ess_volt_out/1, [ess_plant_volt_out_simu]
  1\ess.plant.init.num_module_parallel1/1 -> ess_cell/1(ess_cell_curr)  "ess_cell_curr"
  ess_cell/1(ess_cell_volt_out) -> "ess.plant.init.num_cell_series "/1
  [ess_plant_curr_pol2_simu] -> ess_plant_curr_pol2_simu/1  "ess_plant_curr_pol2_simu"
  [ess_plant_curr_pol1_simu] -> ess_plant_curr_pol1_simu/1  "ess_plant_curr_pol1_simu"
  [ess_plant_rpol2_simu] -> ess_plant_rpol2_simu/1  "ess_plant_rpol2_simu"
  [ess_plant_rpol1_simu] -> ess_plant_rpol1_simu/1  "ess_plant_rpol1_simu"
  [ess_plant_rint_simu] -> ess_plant_rint_simu/1  "ess_plant_rint_simu"
  [ess_plant_voc_simu] -> ess_plant_voc_simu/1  "ess_plant_voc_simu"
  [ess_plant_volt_out_simu] -> ess_plant_volt_out_simu/1  "ess_plant_volt_out_simu"
  [ess_plant_curr_out_simu] -> ess_plant_curr_out_simu/1  "ess_plant_curr_out_simu"
  [ess_plant_soc_simu] -> ess_plant_soc_simu/1  "ess_plant_soc_simu"
  ess_volt_in/1 -> Terminator2/1
  Ground/1 -> ess_curr_in/1
